simulink model "robotwithwall1"  (R2021b)
settings: Solver=FixedStepAuto  StartTime=0.0  StopTime=5  FixedStep=1e-3  RelTol=1e-3
values from neighbouring files (symbols this model uses):
  Bdes = 20    [simIRB120wall.m]    (also in simIRB120wall_fixedTdes.m)
  fdes = 2.5    [simIRB120wall.m]    (also in simIRB120wall_fixedTdes.m)
  kd = [3;3;3;5;5;5]    [simIRB120wall.m]    (also in simIRB120wall_fixedTdes.m)
  ki = [.1;.5;.2;.1;.1;.1]    [simIRB120wall.m]    (also in simIRB120wall_fixedTdes.m)
  kp = [5;5;5;5;5;5]    [simIRB120wall.m]    (also in simIRB120wall_fixedTdes.m)
  kspring = 20    [simIRB120wall.m]    (also in simIRB120wall_fixedTdes.m)
  qdotinit = zeros(6,1)    [simIRB120wall.m]    (also in simIRB120wall_fixedTdes.m)
  qinit = zeros(6,1)    [simIRB120wall.m]    (also in simIRB120wall_fixedTdes.m)
  Tdes = [eye(3,3) [0.5;0;0.5];0 0 0 1]    [simIRB120wall.m]    (also in simIRB120wall_fixedTdes.m = [eye(3,3) [0.7;0;0.5];0 0 0 1])
  x = [-17.0122   -3.0550   -5.6141    0.0007   -0.0846   -3.0546   -5.6091      0.0796   -0.0812    0.0848    0.0814   -0.0814]'    [simIRB120wall.m]    (also in simIRB120wall_fixedTdes.m)
  xwall = 0.5    [simIRB120wall.m]    (also in simIRB120wall_fixedTdes.m)
libraries: robotmaniplib x3, slpidlib x1
settings Model: Creator=wen  LastModifiedBy=wen
settings SolverCC: AlgebraicLoopSolver=TrustRegion
settings DebuggingCC: SFMachineParentedDataDiag=warning

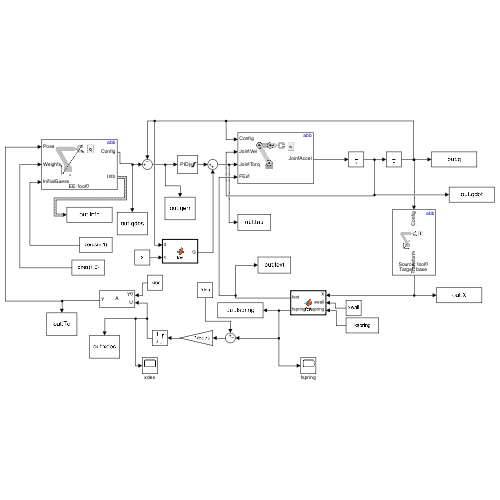
[thumbnail: Simulink's stored preview of the top-level diagram]
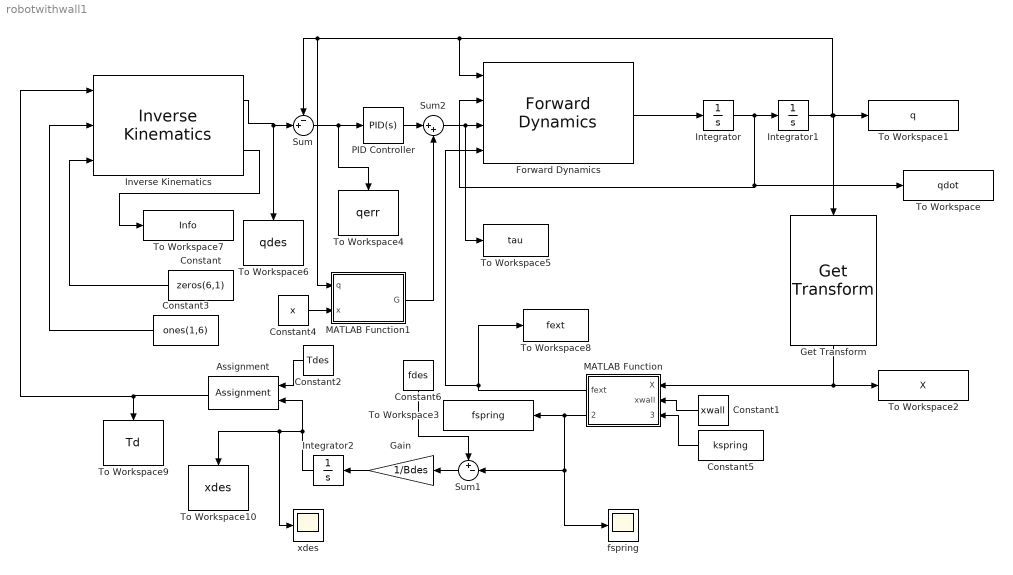
== system robotwithwall1 ==
  Assignment : Assignment  NumberOfDimensions=2  DiagnosticForDimensions=Warning  IndexOptions=Index vector (dialog),Index vector (dialog)  Indices=1,4  OutputSizes=1,1
  Constant : Constant  Value=zeros(6,1)
  Constant1 : Constant  Value=xwall
  Constant2 : Constant  Value=Tdes
  Constant3 : Constant  Value=ones(1,6)
  Constant4 : Constant  Value=x
  Constant5 : Constant  Value=kspring
  Constant6 : Constant  Value=fdes
  Forward Dynamics : robotmaniplib/Forward Dynamics  RigidBodyTree=abb  SimulateUsing=Interpreted execution
  Gain : Gain  Gain=1/Bdes
  Get Transform : robotmaniplib/Get Transform  RigidBodyTree=abb  SourceBody=tool0  TargetBody=base  SimulateUsing=Interpreted execution
  Integrator : Integrator  InitialCondition=qdotinit
  Integrator1 : Integrator  InitialCondition=qinit
  Integrator2 : Integrator  InitialCondition=xwall  LimitOutput=on  UpperSaturationLimit=100
  Inverse Kinematics : robotmaniplib/Inverse Kinematics  RigidBodyTree=abb  EndEffector=tool0  ShowInfo=on  SolverName=BFGS Gradient Projection  EnforceJointLimits=on  MaxIterations=1500  MaxTime=10  GradientTolerance=1e-7  SolutionTolerance=1e-6  StepTolerance=1e-14  ErrorChangeTolerance=1e-12  UseErrorDamping=on  DampingBias=0.0025  SimulateUsing=Interpreted execution
  MATLAB Function : MATLAB Function  TreatAsAtomicUnit=on
  MATLAB Function1 : MATLAB Function  TreatAsAtomicUnit=on
  PID Controller : slpidlib/PID Controller  Controller=PID  Form=Parallel  TimeDomain=Continuous-time  UseExternalTs=off  SampleTime=-1  IntegratorMethod=Forward Euler  FilterMethod=Forward Euler  ControllerParametersSource=internal  P=kp  I=ki  D=kd  UseFilter=on  N=100  TunerSelectOption=Transfer Function Based (PID Tuner App)  InitialConditionSource=internal  InitialConditionForIntegrator=0  InitialConditionForFilter=0  DifferentiatorICPrevScaledInput=0  ExternalReset=none  TrackingMode=off  Kt=1  LimitOutput=on  SatLimitsSource=internal  UpperSaturationLimit=[20;20;20;5;5;5]*.5  LowerSaturationLimit=-[20;20;20;5;5;5]*.5  LinearizeAsGain=on  AntiWindupMode=none  Kb=1  POutMin=[]  POutMax=[]  IOutMin=[]  IOutMax=[]  DOutMin=[]  DOutMax=[]  NOutMin=[]  NOutMax=[]  SumOutMin=[]  SumOutMax=[]  SaturationOutMin=[]  SaturationOutMax=[]  PParamMin=[]  PParamMax=[]  IParamMin=[]  IParamMax=[]  DParamMin=[]  DParamMax=[]  NParamMin=[]  NParamMax=[]  KbParamMin=[]  KbParamMax=[]  KtParamMin=[]  KtParamMax=[]  KbOutMin=[]  KbOutMax=[]  KtOutMin=[]  KtOutMax=[]  IntegratorOutMin=[]  IntegratorOutMax=[]  FilterOutMin=[]  FilterOutMax=[]  SumI1OutMin=[]  SumI1OutMax=[]  SumI2OutMin=[]  SumI2OutMax=[]  SumI3OutMin=[]  SumI3OutMax=[]  SumI4OutMin=[]  SumI4OutMax=[]  SumDOutMin=[]  SumDOutMax=[]  DifferentiatorOutMin=[]  DifferentiatorOutMax=[]  FilterDiffOutCoefMin=[]  FilterDiffOutCoefMax=[]  ReciprocalOutMin=[]  ReciprocalOutMax=[]  SumDenOutMin=[]  SumDenOutMax=[]  SumNumOutMin=[]  SumNumOutMax=[]  DivideOutMin=[]  DivideOutMax=[]  UdiffTsProdOutMin=[]  UdiffTsProdOutMax=[]  NTsProdOutMin=[]  NTsProdOutMax=[]  UintegralTsProdOutMin=[]  UintegralTsProdOutMax=[]  UngainTsProdOutMin=[]  UngainTsProdOutMax=[]  IntegratorContinuousStateAttributes=''  IntegratorStateMustResolveToSignalObject=off  IntegratorRTWStateStorageClass=Auto  FilterContinuousStateAttributes=''  FilterStateMustResolveToSignalObject=off  FilterRTWStateStorageClass=Auto  ParallelPVariant=InternalParameters  IdealPVariant=Disabled  IVariant=InternalParameters  DVariant=InternalParameters  IntegratorVariant=Continuous  SatVariant=Enabled  AWVariant=Passthrough  PCopyVariant=Disabled  TRVariant=Disabled  FdbkBlocksVariant=Forward  IdealPFdbkVariant=Disabled  SatFdbkVariant=Disabled  DerivativeFilterVariant=ContFilter  NVariant=InternalParameters  NCopyVariant=Disabled  FilterICVariant=InternalICsFilter  IntegratorICVariant=InternalICs  ExternalResetVariant=Disabled  TRSumVariant=Passthrough  SumFdbkVariant=Disabled  SumVariant=Sum_PID  TsampFilterVariant=InternalTs  TsampNgainVariant=Passthrough  TsampIntegralVariant=Passthrough  ExternalSaturationOutDataTypeStr=Inherit: Same as second input
  Sum : Sum  Inputs=-+|
  Sum1 : Sum  Inputs=+-|
  Sum2 : Sum  Inputs=|++
  To Workspace : ToWorkspace  VariableName=qdot  SampleTime=-1
  To Workspace1 : ToWorkspace  VariableName=q  SampleTime=-1
  To Workspace10 : ToWorkspace  VariableName=xdes  SaveFormat=Structure With Time  SampleTime=-1
  To Workspace2 : ToWorkspace  VariableName=X  SampleTime=-1
  To Workspace3 : ToWorkspace  VariableName=fspring  SampleTime=-1
  To Workspace4 : ToWorkspace  VariableName=qerr  SampleTime=-1
  To Workspace5 : ToWorkspace  VariableName=tau  SampleTime=-1
  To Workspace6 : ToWorkspace  VariableName=qdes  SampleTime=-1
  To Workspace7 : ToWorkspace  VariableName=Info  SaveFormat=Timeseries  SampleTime=-1
  To Workspace8 : ToWorkspace  VariableName=fext  SampleTime=-1
  To Workspace9 : ToWorkspace  VariableName=Td  SampleTime=-1
  fspring : Scope
  xdes : Scope
  wires:
  Forward Dynamics/1 -> Integrator/1
  Integrator/1 -> Forward Dynamics/2, To Workspace/1, Integrator1/1
  Integrator1/1 -> To Workspace1/1, Get Transform/1, MATLAB Function1/1(q), Sum/1, Forward Dynamics/1
  Sum2/1 -> To Workspace5/1, Forward Dynamics/3
  MATLAB Function/1(fext) -> To Workspace8/1, Forward Dynamics/4
  Sum/1 -> To Workspace4/1, PID Controller/1
  PID Controller/1 -> Sum2/1
  Get Transform/1 -> MATLAB Function/1(X), To Workspace2/1
  Constant1/1 -> MATLAB Function/2(xwall)
  Constant/1 -> Inverse Kinematics/3
  Constant3/1 -> Inverse Kinematics/2
  Inverse Kinematics/1 -> Sum/2, To Workspace6/1
  Constant4/1 -> MATLAB Function1/2(x)
  MATLAB Function1/1(G) -> Sum2/2
  Assignment/1 -> Inverse Kinematics/1, To Workspace9/1
  Inverse Kinematics/2 -> To Workspace7/1
  Constant5/1 -> MATLAB Function/3(kspring)
  MATLAB Function/2(fspring) -> fspring/1, Sum1/2, To Workspace3/1
  Constant2/1 -> Assignment/1
  Constant6/1 -> Sum1/1
  Sum1/1 -> Gain/1
  Gain/1 -> Integrator2/1
  Integrator2/1 -> xdes/1, To Workspace10/1, Assignment/2

== matlab function robotwithwall1/MATLAB Function1 ==
  data: q input; G output; x input
function G = fcn(q,x)

s2=sin(q(2));
s23=sin(q(2)+q(3));
c23=cos(q(2)+q(3));
s4=sin(q(4));
c4=cos(q(4));
s5=sin(q(5));
c5=cos(q(5));

nx=12;
Aq=[zeros(1,nx);
    s2 s23 c23 s23*c4*s5 c23*c5 zeros(1,nx-5);...
    zeros(1,5) s23 c23 s23*c4*s5 c23*c5 zeros(1,nx-9);...
    zeros(1,9) c23*s4*s5 zeros(1,nx-10);...
    zeros(1,10) s23*s5 c23*c4*c5;...
    zeros(1,nx)];

G = Aq*x;

end

== matlab function robotwithwall1/MATLAB Function ==
  data: X input; fext output; xwall input; fspring output; kspring input
function [fext,fspring] = fcn(X,xwall,kspring)

fspring=0;
if (X(1,4)>xwall)
  fspring=kspring*(X(1,4)-xwall);
end
fext=zeros(6,8);
fext(1,8)=fspring;

end
